simulink model "RadioReceiver_FP_clean"  (R2017a)
settings: Solver=FixedStepDiscrete  StartTime=0.0  StopTime=10.0  RelTol=1e-3
InitFcn:
  | barker = comm.BarkerCode('SamplesPerFrame', 28, 'Length', 11);
  | seq = barker()+1;
  | M = 4;
  | hPSKModTrain   = comm.PSKModulator(M, ...
  |     'PhaseOffset',pi/4, ...
  |     'SymbolMapping','Binary');
  | xPreambleSeq = hPSKModTrain(seq);
  | 
  | 
  | %%%%%%%%%%%%
  | 
  | % AGC Preamble
  | reps = 5;
  | barker = comm.BarkerCode('SamplesPerFrame', 16, 'Length', 13);
  | seq = barker()+1;
  | %preamble = zeros(16*reps,1);
  | preambleFull = repmat(seq,reps,1);
  | rctFilt = comm.RaisedCosineTransmitFilter('FilterSpanInSymbols', 128,...
  | 'RolloffFactor',0.5,...
  | 'OutputSamplesPerSymbol',4);
  | preambleFullFilt = rctFilt(preambleFull);
  | 
  | %%%%%%%%%%%%
  | 
  | RadioSampleRate = 1e6;
  | RadioFrameLength = 1e5;
  | 
  | VibertiTracebackLength = 34+20;
  | numTrainingSamples = 250;
  | crc32Poly = [1 0 0 0 0 0 1 0 0 1 1 0 0 0 0 0 1 0 0 0 1 1 1 0 1 1 0 1 1 0 1 1 1];
  | crcDecodeLag = length(crc32Poly)+2;
  | 
  | %%%%%%%%%%%%
  | 
  | beta = 0.5;
  | span = 8;
  | sps = 4;
  | filterGain = 1;
  | coeff = rcosdesign(beta, span, sps, 'sqrt')*filterGain;
  | 
  | %%%%%%%%%%%%
  | 
  | samplesPerSymbol = 4;
  | maxPacketBits = 8*1500;
  | bItsPerSymbol = 2;
  | CodeRate = 2;
  | tailSymbols = 40;
  | maxPayloadSymbols = maxPacketBits*CodeRate/bItsPerSymbol+tailSymbols;
undefined symbols (not defined in the file or in its folder): F, j
libraries: dsphdlfiltering x20, simulink x7, dspstat3 x2, hdlsllib x2, commdigbbndpm3 x2, commsource2 x1, commcrc2 x1, commseqgen3 x1, commcnvcod2 x1, commutil2 x1, zc706fmc234_lib x1
(part 2 of 3)

== system RadioReceiver_FP_clean/Receiver/Gardner Timing Recovery/Gardner TED Blocks/Real Error ==
  data : Inport
  strobe sum : Inport  Port=2
  Delay : Delay  DelayLength=1
  Product1 : Product  OutDataTypeStr=fixdt(1,16,13)
  Sub : Sum  Inputs=+-  AccumDataTypeStr=fixdt(1,16,13)
  TED Buffer Update1 : Subsystem
  Out1 : Outport
  wires:
  Product1/1 -> Out1/1
  Sub/1 -> Product1/2
  data/1 -> Sub/2, Delay/1
  strobe sum/1 -> TED Buffer Update1/2(strobe sum)
  TED Buffer Update1/2(oldest) -> Sub/1
  Delay/1 -> TED Buffer Update1/1(new data)
  TED Buffer Update1/1(Middle Indx) -> Product1/1

== system RadioReceiver_FP_clean/Receiver/Gardner Timing Recovery/Gardner TED Blocks (NBS)/Imag Error ==
  data : Inport
  strobe sum : Inport  Port=2
  Delay : Delay  DelayLength=1
  Product1 : Product  OutDataTypeStr=fixdt(1,16,13)
  Sub : Sum  Inputs=+-  AccumDataTypeStr=fixdt(1,16,13)
  TED Buffer Update1 : Subsystem
  Out1 : Outport
  wires:
  Product1/1 -> Out1/1
  Sub/1 -> Product1/2
  data/1 -> Sub/2, Delay/1
  strobe sum/1 -> TED Buffer Update1/2(strobe sum)
  TED Buffer Update1/2(oldest) -> Sub/1
  Delay/1 -> TED Buffer Update1/1(new data)
  TED Buffer Update1/1(Middle Indx) -> Product1/1

== system RadioReceiver_FP_clean/Receiver/Gardner Timing Recovery/Gardner TED Blocks (NBS)/Real Error ==
  data : Inport
  strobe sum : Inport  Port=2
  Delay : Delay  DelayLength=1
  Product1 : Product  OutDataTypeStr=fixdt(1,16,13)
  Sub : Sum  Inputs=+-  AccumDataTypeStr=fixdt(1,16,13)
  TED Buffer Update1 : Subsystem
  Out1 : Outport
  wires:
  Product1/1 -> Out1/1
  Sub/1 -> Product1/2
  data/1 -> Sub/2, Delay/1
  strobe sum/1 -> TED Buffer Update1/2(strobe sum)
  TED Buffer Update1/2(oldest) -> Sub/1
  Delay/1 -> TED Buffer Update1/1(new data)
  TED Buffer Update1/1(Middle Indx) -> Product1/1

== system RadioReceiver_FP_clean/Receiver/Gardner Timing Recovery/InterpControl_Blocks/Calculate New mu ==
  W : Inport
  NCOCounter : Inport  Port=2
  Math Reciprocal : Math  Operator=reciprocal  RndMeth=Zero  SaturateOnIntegerOverflow=on
  Product : Product  OutDataTypeStr=fixdt(1,14,15)
  mu : Outport
  wires:
  Product/1 -> mu/1
  W/1 -> Math Reciprocal/1
  Math Reciprocal/1 -> Product/1
  NCOCounter/1 -> Product/2

== system RadioReceiver_FP_clean/Receiver/Frame Sync and Decode/Barker Locate/Measure Phase Ambiguity/Find Max and Set Output Shift ==
  In1 : Inport  OutDataTypeStr=int16
  In2 : Inport  Port=2  OutDataTypeStr=int16
  In4 : Inport  Port=3  OutDataTypeStr=int16
  In5 : Inport  Port=4  OutDataTypeStr=int16
  Enable : EnablePort
  Complex to Real-Imag{,1..3} (4 alike) : ComplexToRealImag  Output=Imag
  Direct Lookup Table (n-D) : LookupNDDirect  NumberOfTableDimensions=1  Table=exp(-(0:pi/2:(pi*3/2)) .* 1i).'  DiagnosticForOutOfRangeInput=Error  TableDataTypeStr=fixdt(1,16,13)
  Maximum : dspstat3/Maximum  operation=maximum  fcn=Index  indexBase=Zero  operateOver=Each column  Dimension=1  InputProcessing=Columns as channels (frame based)  reset=None  roiEnable=off  roiType=Rectangles  roiPortion=Entire ROI  roiOutput=Individual statistics for each ROI  roiFlag=off  roundingMode=Floor  overflowMode=off  accumDataTypeStr=Inherit: Same as product output  accumLastDataTypeStr=Inherit: Same as product output
  Vector Concatenate : Concatenate  NumInputs=4
  Out1 : Outport  InitialOutput=0
  wires:
  Direct Lookup Table (n-D)/1 -> Out1/1
  In1/1 -> Complex to Real-Imag/1
  Complex to Real-Imag2/1 -> Vector Concatenate/3
  Complex to Real-Imag1/1 -> Vector Concatenate/2
  In5/1 -> Complex to Real-Imag3/1
  Complex to Real-Imag3/1 -> Vector Concatenate/4
  Complex to Real-Imag/1 -> Vector Concatenate/1
  Maximum/1 -> Direct Lookup Table (n-D)/1
  In2/1 -> Complex to Real-Imag1/1
  Vector Concatenate/1 -> Maximum/1
  In4/1 -> Complex to Real-Imag2/1

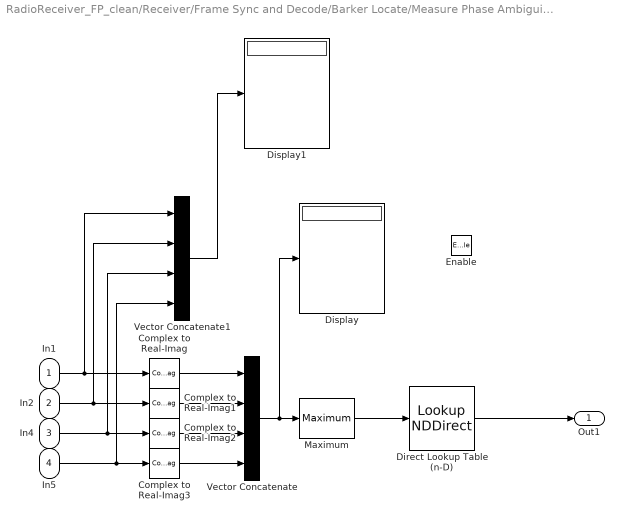
== system RadioReceiver_FP_clean/Receiver/Frame Sync and Decode/Barker Locate/Measure Phase Ambiguity1/Find Max and Set Output Shift ==
  In1 : Inport
  In2 : Inport  Port=2
  In4 : Inport  Port=3
  In5 : Inport  Port=4
  Enable : EnablePort
  Complex to Real-Imag{,1..3} (4 alike) : ComplexToRealImag  Output=Imag
  Direct Lookup Table (n-D) : LookupNDDirect  NumberOfTableDimensions=1  Table=exp(-(0:pi/2:(pi*3/2)) .* 1i).'  DiagnosticForOutOfRangeInput=Error  TableDataTypeStr=fixdt(1,16,13)
  Display : Display
  Display1 : Display
  Maximum : dspstat3/Maximum  operation=maximum  fcn=Index  indexBase=Zero  operateOver=Each column  Dimension=1  InputProcessing=Columns as channels (frame based)  reset=None  roiEnable=off  roiType=Rectangles  roiPortion=Entire ROI  roiOutput=Individual statistics for each ROI  roiFlag=off  roundingMode=Floor  overflowMode=off  accumDataTypeStr=Inherit: Same as product output  accumLastDataTypeStr=Inherit: Same as product output
  Vector Concatenate : Concatenate  NumInputs=4
  Vector Concatenate1 : Concatenate  NumInputs=4
  Out1 : Outport  InitialOutput=0
  wires:
  Direct Lookup Table (n-D)/1 -> Out1/1
  In4/1 -> Vector Concatenate1/3, Complex to Real-Imag2/1
  In2/1 -> Vector Concatenate1/2, Complex to Real-Imag1/1
  In5/1 -> Vector Concatenate1/4, Complex to Real-Imag3/1
  In1/1 -> Vector Concatenate1/1, Complex to Real-Imag/1
  Maximum/1 -> Direct Lookup Table (n-D)/1
  Vector Concatenate/1 -> Display/1, Maximum/1
  Complex to Real-Imag/1 -> Vector Concatenate/1
  Complex to Real-Imag1/1 -> Vector Concatenate/2
  Complex to Real-Imag2/1 -> Vector Concatenate/3
  Complex to Real-Imag3/1 -> Vector Concatenate/4
  Vector Concatenate1/1 -> Display1/1

== system RadioReceiver_FP_clean/Receiver/Frame Sync and Decode/Barker Locate/Measure Phase Ambiguity1/HDL Opt Complex FIR4 ==
  In1 : Inport
  validIn : Inport  Port=2
  Add : Sum  Inputs=+-  AccumDataTypeStr=fixdt(1,16,0)
  Complex to Real-Imag : ComplexToRealImag
  Discrete FIR Filter HDL Optimized : dsphdlfiltering/Discrete FIR Filter HDL Optimized  Numerator=real(Taps)  Sharing=off  SharingFactor=2  SimulateUsing=Code generation  roundingMode=Floor  overflowMode=off  CoefficientsDataTypeStr=Inherit: Same word length as input  CoefficientsMin=[]  CoefficientsMax=[]  OutputDataTypeStr=fixdt(1,16,0)  OutputMin=[]  OutputMax=[]  ValidInPort=on  ReadyPort=off
      settings: SourceProductName=DSP System Toolbox  SourceProductBaseCode=DS
  Discrete FIR Filter HDL Optimized1 : dsphdlfiltering/Discrete FIR Filter HDL Optimized  Numerator=imag(Taps)  Sharing=off  SharingFactor=2  SimulateUsing=Code generation  roundingMode=Floor  overflowMode=off  CoefficientsDataTypeStr=Inherit: Same word length as input  CoefficientsMin=[]  CoefficientsMax=[]  OutputDataTypeStr=fixdt(1,16,0)  OutputMin=[]  OutputMax=[]  ValidInPort=on  ReadyPort=off
      settings: SourceProductName=DSP System Toolbox  SourceProductBaseCode=DS
  Discrete FIR Filter HDL Optimized2 : dsphdlfiltering/Discrete FIR Filter HDL Optimized  Numerator=real(Taps)  Sharing=off  SharingFactor=2  SimulateUsing=Code generation  roundingMode=Floor  overflowMode=off  CoefficientsDataTypeStr=Inherit: Same word length as input  CoefficientsMin=[]  CoefficientsMax=[]  OutputDataTypeStr=fixdt(1,16,0)  OutputMin=[]  OutputMax=[]  ValidInPort=on  ReadyPort=off
      settings: SourceProductName=DSP System Toolbox  SourceProductBaseCode=DS
  Discrete FIR Filter HDL Optimized3 : dsphdlfiltering/Discrete FIR Filter HDL Optimized  Numerator=imag(Taps)  Sharing=off  SharingFactor=2  SimulateUsing=Code generation  roundingMode=Floor  overflowMode=off  CoefficientsDataTypeStr=Inherit: Same word length as input  CoefficientsMin=[]  CoefficientsMax=[]  OutputDataTypeStr=fixdt(1,16,0)  OutputMin=[]  OutputMax=[]  ValidInPort=on  ReadyPort=off
      settings: SourceProductName=DSP System Toolbox  SourceProductBaseCode=DS
  Logical Operator : Logic  Inputs=4  AllPortsSameDT=off  OutDataTypeStr=boolean
  Real-Imag to Complex : RealImagToComplex
  Subtract : Sum  OutDataTypeStr=int16
  Out1 : Outport
  validOut : Outport  Port=2
  wires:
  Discrete FIR Filter HDL Optimized/1 -> Add/1
  Logical Operator/1 -> validOut/1
  Discrete FIR Filter HDL Optimized/2 -> Logical Operator/1
  Discrete FIR Filter HDL Optimized1/2 -> Logical Operator/2
  Discrete FIR Filter HDL Optimized1/1 -> Add/2
  validIn/1 -> Discrete FIR Filter HDL Optimized3/2, Discrete FIR Filter HDL Optimized2/2, Discrete FIR Filter HDL Optimized1/2, Discrete FIR Filter HDL Optimized/2
  In1/1 -> Complex to Real-Imag/1
  Complex to Real-Imag/1 -> Discrete FIR Filter HDL Optimized3/1, Discrete FIR Filter HDL Optimized/1
  Discrete FIR Filter HDL Optimized2/2 -> Logical Operator/3
  Discrete FIR Filter HDL Optimized3/2 -> Logical Operator/4
  Complex to Real-Imag/2 -> Discrete FIR Filter HDL Optimized2/1, Discrete FIR Filter HDL Optimized1/1
  Discrete FIR Filter HDL Optimized2/1 -> Subtract/1
  Discrete FIR Filter HDL Optimized3/1 -> Subtract/2
  Real-Imag to Complex/1 -> Out1/1
  Subtract/1 -> Real-Imag to Complex/2
  Add/1 -> Real-Imag to Complex/1

== system RadioReceiver_FP_clean/Receiver/Frame Sync and Decode/Barker Locate/Measure Phase Ambiguity1/HDL Opt Complex FIR5 ==
  In1 : Inport
  validIn : Inport  Port=2
  Add : Sum  Inputs=+-  AccumDataTypeStr=fixdt(1,16,0)
  Complex to Real-Imag : ComplexToRealImag
  Discrete FIR Filter HDL Optimized : dsphdlfiltering/Discrete FIR Filter HDL Optimized  Numerator=real(Taps)  Sharing=off  SharingFactor=2  SimulateUsing=Code generation  roundingMode=Floor  overflowMode=off  CoefficientsDataTypeStr=Inherit: Same word length as input  CoefficientsMin=[]  CoefficientsMax=[]  OutputDataTypeStr=fixdt(1,16,0)  OutputMin=[]  OutputMax=[]  ValidInPort=on  ReadyPort=off
      settings: SourceProductName=DSP System Toolbox  SourceProductBaseCode=DS
  Discrete FIR Filter HDL Optimized1 : dsphdlfiltering/Discrete FIR Filter HDL Optimized  Numerator=imag(Taps)  Sharing=off  SharingFactor=2  SimulateUsing=Code generation  roundingMode=Floor  overflowMode=off  CoefficientsDataTypeStr=Inherit: Same word length as input  CoefficientsMin=[]  CoefficientsMax=[]  OutputDataTypeStr=fixdt(1,16,0)  OutputMin=[]  OutputMax=[]  ValidInPort=on  ReadyPort=off
      settings: SourceProductName=DSP System Toolbox  SourceProductBaseCode=DS
  Discrete FIR Filter HDL Optimized2 : dsphdlfiltering/Discrete FIR Filter HDL Optimized  Numerator=real(Taps)  Sharing=off  SharingFactor=2  SimulateUsing=Code generation  roundingMode=Floor  overflowMode=off  CoefficientsDataTypeStr=Inherit: Same word length as input  CoefficientsMin=[]  CoefficientsMax=[]  OutputDataTypeStr=fixdt(1,16,0)  OutputMin=[]  OutputMax=[]  ValidInPort=on  ReadyPort=off
      settings: SourceProductName=DSP System Toolbox  SourceProductBaseCode=DS
  Discrete FIR Filter HDL Optimized3 : dsphdlfiltering/Discrete FIR Filter HDL Optimized  Numerator=imag(Taps)  Sharing=off  SharingFactor=2  SimulateUsing=Code generation  roundingMode=Floor  overflowMode=off  CoefficientsDataTypeStr=Inherit: Same word length as input  CoefficientsMin=[]  CoefficientsMax=[]  OutputDataTypeStr=fixdt(1,16,0)  OutputMin=[]  OutputMax=[]  ValidInPort=on  ReadyPort=off
      settings: SourceProductName=DSP System Toolbox  SourceProductBaseCode=DS
  Logical Operator : Logic  Inputs=4  AllPortsSameDT=off  OutDataTypeStr=boolean
  Real-Imag to Complex : RealImagToComplex
  Subtract : Sum  OutDataTypeStr=int16
  Out1 : Outport
  validOut : Outport  Port=2
  wires:
  Discrete FIR Filter HDL Optimized/1 -> Add/1
  Logical Operator/1 -> validOut/1
  Discrete FIR Filter HDL Optimized/2 -> Logical Operator/1
  Discrete FIR Filter HDL Optimized1/2 -> Logical Operator/2
  Discrete FIR Filter HDL Optimized1/1 -> Add/2
  validIn/1 -> Discrete FIR Filter HDL Optimized3/2, Discrete FIR Filter HDL Optimized2/2, Discrete FIR Filter HDL Optimized1/2, Discrete FIR Filter HDL Optimized/2
  In1/1 -> Complex to Real-Imag/1
  Complex to Real-Imag/1 -> Discrete FIR Filter HDL Optimized3/1, Discrete FIR Filter HDL Optimized/1
  Discrete FIR Filter HDL Optimized2/2 -> Logical Operator/3
  Discrete FIR Filter HDL Optimized3/2 -> Logical Operator/4
  Complex to Real-Imag/2 -> Discrete FIR Filter HDL Optimized2/1, Discrete FIR Filter HDL Optimized1/1
  Discrete FIR Filter HDL Optimized2/1 -> Subtract/1
  Discrete FIR Filter HDL Optimized3/1 -> Subtract/2
  Real-Imag to Complex/1 -> Out1/1
  Subtract/1 -> Real-Imag to Complex/2
  Add/1 -> Real-Imag to Complex/1

== system RadioReceiver_FP_clean/Receiver/Frame Sync and Decode/Barker Locate/Measure Phase Ambiguity1/HDL Opt Complex FIR6 ==
  In1 : Inport
  validIn : Inport  Port=2
  Add : Sum  Inputs=+-  AccumDataTypeStr=fixdt(1,16,0)
  Complex to Real-Imag : ComplexToRealImag
  Discrete FIR Filter HDL Optimized : dsphdlfiltering/Discrete FIR Filter HDL Optimized  Numerator=real(Taps)  Sharing=off  SharingFactor=2  SimulateUsing=Code generation  roundingMode=Floor  overflowMode=off  CoefficientsDataTypeStr=Inherit: Same word length as input  CoefficientsMin=[]  CoefficientsMax=[]  OutputDataTypeStr=fixdt(1,16,0)  OutputMin=[]  OutputMax=[]  ValidInPort=on  ReadyPort=off
      settings: SourceProductName=DSP System Toolbox  SourceProductBaseCode=DS
  Discrete FIR Filter HDL Optimized1 : dsphdlfiltering/Discrete FIR Filter HDL Optimized  Numerator=imag(Taps)  Sharing=off  SharingFactor=2  SimulateUsing=Code generation  roundingMode=Floor  overflowMode=off  CoefficientsDataTypeStr=Inherit: Same word length as input  CoefficientsMin=[]  CoefficientsMax=[]  OutputDataTypeStr=fixdt(1,16,0)  OutputMin=[]  OutputMax=[]  ValidInPort=on  ReadyPort=off
      settings: SourceProductName=DSP System Toolbox  SourceProductBaseCode=DS
  Discrete FIR Filter HDL Optimized2 : dsphdlfiltering/Discrete FIR Filter HDL Optimized  Numerator=real(Taps)  Sharing=off  SharingFactor=2  SimulateUsing=Code generation  roundingMode=Floor  overflowMode=off  CoefficientsDataTypeStr=Inherit: Same word length as input  CoefficientsMin=[]  CoefficientsMax=[]  OutputDataTypeStr=fixdt(1,16,0)  OutputMin=[]  OutputMax=[]  ValidInPort=on  ReadyPort=off
      settings: SourceProductName=DSP System Toolbox  SourceProductBaseCode=DS
  Discrete FIR Filter HDL Optimized3 : dsphdlfiltering/Discrete FIR Filter HDL Optimized  Numerator=imag(Taps)  Sharing=off  SharingFactor=2  SimulateUsing=Code generation  roundingMode=Floor  overflowMode=off  CoefficientsDataTypeStr=Inherit: Same word length as input  CoefficientsMin=[]  CoefficientsMax=[]  OutputDataTypeStr=fixdt(1,16,0)  OutputMin=[]  OutputMax=[]  ValidInPort=on  ReadyPort=off
      settings: SourceProductName=DSP System Toolbox  SourceProductBaseCode=DS
  Logical Operator : Logic  Inputs=4  AllPortsSameDT=off  OutDataTypeStr=boolean
  Real-Imag to Complex : RealImagToComplex
  Subtract : Sum  OutDataTypeStr=int16
  Out1 : Outport
  validOut : Outport  Port=2
  wires:
  Discrete FIR Filter HDL Optimized/1 -> Add/1
  Logical Operator/1 -> validOut/1
  Discrete FIR Filter HDL Optimized/2 -> Logical Operator/1
  Discrete FIR Filter HDL Optimized1/2 -> Logical Operator/2
  Discrete FIR Filter HDL Optimized1/1 -> Add/2
  validIn/1 -> Discrete FIR Filter HDL Optimized3/2, Discrete FIR Filter HDL Optimized2/2, Discrete FIR Filter HDL Optimized1/2, Discrete FIR Filter HDL Optimized/2
  In1/1 -> Complex to Real-Imag/1
  Complex to Real-Imag/1 -> Discrete FIR Filter HDL Optimized3/1, Discrete FIR Filter HDL Optimized/1
  Discrete FIR Filter HDL Optimized2/2 -> Logical Operator/3
  Discrete FIR Filter HDL Optimized3/2 -> Logical Operator/4
  Complex to Real-Imag/2 -> Discrete FIR Filter HDL Optimized2/1, Discrete FIR Filter HDL Optimized1/1
  Discrete FIR Filter HDL Optimized2/1 -> Subtract/1
  Discrete FIR Filter HDL Optimized3/1 -> Subtract/2
  Real-Imag to Complex/1 -> Out1/1
  Subtract/1 -> Real-Imag to Complex/2
  Add/1 -> Real-Imag to Complex/1

== system RadioReceiver_FP_clean/Receiver/Frame Sync and Decode/Barker Locate/Measure Phase Ambiguity1/HDL Opt Complex FIR7 ==
  In1 : Inport
  validIn : Inport  Port=2
  Add : Sum  Inputs=+-  AccumDataTypeStr=fixdt(1,16,0)
  Complex to Real-Imag : ComplexToRealImag
  Discrete FIR Filter HDL Optimized : dsphdlfiltering/Discrete FIR Filter HDL Optimized  Numerator=real(Taps)  Sharing=off  SharingFactor=2  SimulateUsing=Code generation  roundingMode=Floor  overflowMode=off  CoefficientsDataTypeStr=Inherit: Same word length as input  CoefficientsMin=[]  CoefficientsMax=[]  OutputDataTypeStr=fixdt(1,16,0)  OutputMin=[]  OutputMax=[]  ValidInPort=on  ReadyPort=off
      settings: SourceProductName=DSP System Toolbox  SourceProductBaseCode=DS
  Discrete FIR Filter HDL Optimized1 : dsphdlfiltering/Discrete FIR Filter HDL Optimized  Numerator=imag(Taps)  Sharing=off  SharingFactor=2  SimulateUsing=Code generation  roundingMode=Floor  overflowMode=off  CoefficientsDataTypeStr=Inherit: Same word length as input  CoefficientsMin=[]  CoefficientsMax=[]  OutputDataTypeStr=fixdt(1,16,0)  OutputMin=[]  OutputMax=[]  ValidInPort=on  ReadyPort=off
      settings: SourceProductName=DSP System Toolbox  SourceProductBaseCode=DS
  Discrete FIR Filter HDL Optimized2 : dsphdlfiltering/Discrete FIR Filter HDL Optimized  Numerator=real(Taps)  Sharing=off  SharingFactor=2  SimulateUsing=Code generation  roundingMode=Floor  overflowMode=off  CoefficientsDataTypeStr=Inherit: Same word length as input  CoefficientsMin=[]  CoefficientsMax=[]  OutputDataTypeStr=fixdt(1,16,0)  OutputMin=[]  OutputMax=[]  ValidInPort=on  ReadyPort=off
      settings: SourceProductName=DSP System Toolbox  SourceProductBaseCode=DS
  Discrete FIR Filter HDL Optimized3 : dsphdlfiltering/Discrete FIR Filter HDL Optimized  Numerator=imag(Taps)  Sharing=off  SharingFactor=2  SimulateUsing=Code generation  roundingMode=Floor  overflowMode=off  CoefficientsDataTypeStr=Inherit: Same word length as input  CoefficientsMin=[]  CoefficientsMax=[]  OutputDataTypeStr=fixdt(1,16,0)  OutputMin=[]  OutputMax=[]  ValidInPort=on  ReadyPort=off
      settings: SourceProductName=DSP System Toolbox  SourceProductBaseCode=DS
  Logical Operator : Logic  Inputs=4  AllPortsSameDT=off  OutDataTypeStr=boolean
  Real-Imag to Complex : RealImagToComplex
  Subtract : Sum  OutDataTypeStr=int16
  Out1 : Outport
  validOut : Outport  Port=2
  wires:
  Discrete FIR Filter HDL Optimized/1 -> Add/1
  Logical Operator/1 -> validOut/1
  Discrete FIR Filter HDL Optimized/2 -> Logical Operator/1
  Discrete FIR Filter HDL Optimized1/2 -> Logical Operator/2
  Discrete FIR Filter HDL Optimized1/1 -> Add/2
  validIn/1 -> Discrete FIR Filter HDL Optimized3/2, Discrete FIR Filter HDL Optimized2/2, Discrete FIR Filter HDL Optimized1/2, Discrete FIR Filter HDL Optimized/2
  In1/1 -> Complex to Real-Imag/1
  Complex to Real-Imag/1 -> Discrete FIR Filter HDL Optimized3/1, Discrete FIR Filter HDL Optimized/1
  Discrete FIR Filter HDL Optimized2/2 -> Logical Operator/3
  Discrete FIR Filter HDL Optimized3/2 -> Logical Operator/4
  Complex to Real-Imag/2 -> Discrete FIR Filter HDL Optimized2/1, Discrete FIR Filter HDL Optimized1/1
  Discrete FIR Filter HDL Optimized2/1 -> Subtract/1
  Discrete FIR Filter HDL Optimized3/1 -> Subtract/2
  Real-Imag to Complex/1 -> Out1/1
  Subtract/1 -> Real-Imag to Complex/2
  Add/1 -> Real-Imag to Complex/1

== system RadioReceiver_FP_clean/Receiver/Frame Sync and Decode/Equalization and Demodulation/DFE/Packeted To Unpacked ==
  In1 : Inport
  Extract Bits : simulink/Logic and Bit Operations/Extract Bits  bitsToExtract=Range of bits  numBits=8  bitIdxRange=[1]  outScalingMode=Treat bit field as an integer
      settings: SourceProductName=Simulink
  Extract Bits1 : simulink/Logic and Bit Operations/Extract Bits  bitsToExtract=Range of bits  numBits=8  bitIdxRange=[0]  outScalingMode=Treat bit field as an integer
      settings: SourceProductName=Simulink
  Vector Concatenate : Concatenate
  Out1 : Outport
  wires:
  In1/1 -> Extract Bits1/1, Extract Bits/1
  Extract Bits/1 -> Vector Concatenate/1
  Extract Bits1/1 -> Vector Concatenate/2
  Vector Concatenate/1 -> Out1/1

== system RadioReceiver_FP_clean/Receiver/Frame Sync and Decode/Equalization and Demodulation/DMA Interface/Convert Payload Length To Bytes ==
  In1 : Inport
  Constant : Constant  Value=uint16(32-1)  SampleTime=-1
  Data Type Conversion : DataTypeConversion  OutDataTypeStr=uint32
  Remove CRC Length : Sum  Inputs=+-  AccumDataTypeStr=uint16
  Shift Arithmetic1 : ArithShift  BitShiftNumber=3  BitShiftDirection=Right
  Shift Arithmetic2 : ArithShift  BitShiftNumber=1  BitShiftDirection=Right
  Out1 : Outport
  wires:
  In1/1 -> Shift Arithmetic2/1
  Remove CRC Length/1 -> Shift Arithmetic1/1
  Shift Arithmetic2/1 -> Remove CRC Length/1
  Shift Arithmetic1/1 -> Data Type Conversion/1
  Constant/1 -> Remove CRC Length/2
  Data Type Conversion/1 -> Out1/1

== system RadioReceiver_FP_clean/Receiver/Frame Sync and Decode/Equalization and Demodulation/Descramble and Decode/2 Bit Descrambler ==
  note: This is a special Descrambler which can process 2 bits at a time
  u1 : Inport
  reset : Inport  Port=2
  Demux1 : Demux  Outputs=2
  MATLAB Function : MATLAB Function  TreatAsAtomicUnit=on
  Mux : Mux  Inputs=2
  Selector1 : Selector  IndexOptions=Index vector (dialog)  Indices=find(polynom(2:end))  OutputSizes=1
  Selector2 : Selector  IndexOptions=Index vector (dialog)  Indices=find(polynom(2:end))  OutputSizes=1
  input_xor1 : Logic  Operator=XOR  IconShape=distinctive  AllPortsSameDT=off  OutDataTypeStr=boolean
  input_xor2 : Logic  Operator=XOR  IconShape=distinctive  AllPortsSameDT=off  OutDataTypeStr=boolean
  state_xor1 : Logic  Operator=XOR  Inputs=1  IconShape=distinctive  AllPortsSameDT=off  OutDataTypeStr=boolean
  state_xor2 : Logic  Operator=XOR  Inputs=1  IconShape=distinctive  AllPortsSameDT=off  OutDataTypeStr=boolean
  y1 : Outport  InitialOutput=0
  wires:
  u1/1 -> Demux1/1, MATLAB Function/1(bits)
  reset/1 -> MATLAB Function/2(reset)
  MATLAB Function/1(bufferA) -> Selector1/1
  MATLAB Function/2(bufferB) -> Selector2/1
  Mux/1 -> y1/1
  state_xor1/1 -> input_xor1/1
  state_xor2/1 -> input_xor2/1
  input_xor2/1 -> Mux/2
  input_xor1/1 -> Mux/1
  Selector1/1 -> state_xor1/1
  Selector2/1 -> state_xor2/1
  Demux1/1 -> input_xor1/2
  Demux1/2 -> input_xor2/2  "data_in"

== system RadioReceiver_FP_clean/Receiver/Frame Sync and Decode/Equalization and Demodulation/Descramble and Decode/Enabled Subsystem ==
  In1 : Inport
  Enable : EnablePort
  To Workspace : ToWorkspace  VariableName=crcConditions  SaveFormat=Structure  SampleTime=-1
  wires:
  In1/1 -> To Workspace/1

== system RadioReceiver_FP_clean/Receiver/Gardner Timing Recovery/Gardner TED Blocks/Imag Error/TED Buffer Update1 ==
  new data : Inport
  strobe sum : Inport  Port=2
  Delay{,1..3} (4 alike) : Delay  DelayLength=1
  Multiport Switch{,1..3} (4 alike) : MultiPortSwitch  DataPortOrder=Zero-based contiguous  DataPortIndices={0,1,[2,3]}
  Zero bit : Constant  Value=0  OutDataTypeStr=fixdt(1,16,13)  SampleTime=1e-6
  Middle Indx : Outport
  oldest : Outport  Port=2
  wires:
  strobe sum/1 -> Multiport Switch3/1, Multiport Switch2/1, Multiport Switch1/1, Multiport Switch/1
  Delay/1 -> Multiport Switch/2
  Delay1/1 -> Multiport Switch/3, Multiport Switch1/2
  Delay2/1 -> Multiport Switch/4, Multiport Switch1/3, Multiport Switch2/2
  new data/1 -> Multiport Switch3/4, Multiport Switch3/3
  Zero bit/1 -> Multiport Switch2/4
  Delay3/1 -> Multiport Switch1/4, Multiport Switch2/3, Multiport Switch3/2
  Multiport Switch1/1 -> Delay1/1
  Multiport Switch2/1 -> Middle Indx/1, Delay2/1
  Multiport Switch3/1 -> Delay3/1
  Multiport Switch/1 -> Delay/1, oldest/1

== system RadioReceiver_FP_clean/Receiver/Gardner Timing Recovery/Gardner TED Blocks/Real Error/TED Buffer Update1 ==
  new data : Inport
  strobe sum : Inport  Port=2
  Delay{,1..3} (4 alike) : Delay  DelayLength=1
  Multiport Switch{,1..3} (4 alike) : MultiPortSwitch  DataPortOrder=Zero-based contiguous  DataPortIndices={0,1,[2,3]}
  Zero bit : Constant  Value=0  OutDataTypeStr=fixdt(1,16,13)  SampleTime=1e-6
  Middle Indx : Outport
  oldest : Outport  Port=2
  wires:
  strobe sum/1 -> Multiport Switch3/1, Multiport Switch2/1, Multiport Switch1/1, Multiport Switch/1
  Delay/1 -> Multiport Switch/2
  Delay1/1 -> Multiport Switch/3, Multiport Switch1/2
  Delay2/1 -> Multiport Switch/4, Multiport Switch1/3, Multiport Switch2/2
  new data/1 -> Multiport Switch3/4, Multiport Switch3/3
  Zero bit/1 -> Multiport Switch2/4
  Delay3/1 -> Multiport Switch1/4, Multiport Switch2/3, Multiport Switch3/2
  Multiport Switch1/1 -> Delay1/1
  Multiport Switch2/1 -> Middle Indx/1, Delay2/1
  Multiport Switch3/1 -> Delay3/1
  Multiport Switch/1 -> Delay/1, oldest/1

== system RadioReceiver_FP_clean/Receiver/Gardner Timing Recovery/Gardner TED Blocks (NBS)/Imag Error/TED Buffer Update1 ==
  new data : Inport
  strobe sum : Inport  Port=2
  Delay{,1..3} (4 alike) : Delay  DelayLength=1
  Multiport Switch{,1..3} (4 alike) : MultiPortSwitch  DataPortOrder=Zero-based contiguous  DataPortIndices={0,1,[2,3]}
  Zero bit : Constant  Value=0  OutDataTypeStr=fixdt(1,16,13)  SampleTime=1e-6
  Middle Indx : Outport
  oldest : Outport  Port=2
  wires:
  strobe sum/1 -> Multiport Switch3/1, Multiport Switch2/1, Multiport Switch1/1, Multiport Switch/1
  Delay/1 -> Multiport Switch/2
  Delay1/1 -> Multiport Switch/3, Multiport Switch1/2
  Delay2/1 -> Multiport Switch/4, Multiport Switch1/3, Multiport Switch2/2
  new data/1 -> Multiport Switch3/4, Multiport Switch3/3
  Zero bit/1 -> Multiport Switch2/4
  Delay3/1 -> Multiport Switch1/4, Multiport Switch2/3, Multiport Switch3/2
  Multiport Switch1/1 -> Delay1/1
  Multiport Switch2/1 -> Middle Indx/1, Delay2/1
  Multiport Switch3/1 -> Delay3/1
  Multiport Switch/1 -> Delay/1, oldest/1

== system RadioReceiver_FP_clean/Receiver/Gardner Timing Recovery/Gardner TED Blocks (NBS)/Real Error/TED Buffer Update1 ==
  new data : Inport
  strobe sum : Inport  Port=2
  Delay{,1..3} (4 alike) : Delay  DelayLength=1
  Multiport Switch{,1..3} (4 alike) : MultiPortSwitch  DataPortOrder=Zero-based contiguous  DataPortIndices={0,1,[2,3]}
  Zero bit : Constant  Value=0  OutDataTypeStr=fixdt(1,16,13)  SampleTime=1e-6
  Middle Indx : Outport
  oldest : Outport  Port=2
  wires:
  strobe sum/1 -> Multiport Switch3/1, Multiport Switch2/1, Multiport Switch1/1, Multiport Switch/1
  Delay/1 -> Multiport Switch/2
  Delay1/1 -> Multiport Switch/3, Multiport Switch1/2
  Delay2/1 -> Multiport Switch/4, Multiport Switch1/3, Multiport Switch2/2
  new data/1 -> Multiport Switch3/4, Multiport Switch3/3
  Zero bit/1 -> Multiport Switch2/4
  Delay3/1 -> Multiport Switch1/4, Multiport Switch2/3, Multiport Switch3/2
  Multiport Switch1/1 -> Delay1/1
  Multiport Switch2/1 -> Middle Indx/1, Delay2/1
  Multiport Switch3/1 -> Delay3/1
  Multiport Switch/1 -> Delay/1, oldest/1

== matlab function RadioReceiver_FP_clean/Receiver/Frame Sync and Decode/Equalization and Demodulation/CRC Check/Check CRC Result (DEBUG) ==
  data: bits input; start input; done input; valid input; err input
function fcn(bits, start, done, valid, err)

persistent buffer

if isempty(buffer)
    buffer = fi(false(1032,1),0,1,0);
end

buffer = [buffer(2:end);bits];

if done && valid
    if err
        fprintf('CRC Error (HDL CRC)\n');
    else
        fprintf('CRC Passed (HDL CRC)\n');
    end
end
if err % Flag if any error every occurs
    fprintf('CRC Error Type 2 (HDL CRC)\n');
end

== matlab function RadioReceiver_FP_clean/Receiver/Gardner Timing Recovery/Gardner TED/Gardner TED ==
  data: u input; strobe input; e output
% function e = TED(u,strobe)
% 
% persistent TEDBuffer StrobeHistory t1Indx t2Indx
% 
% if isempty(TEDBuffer)
%     samplesPerSymbol = 4;
%     TEDBuffer = complex(zeros(samplesPerSymbol,1));
%     StrobeHistory = false(samplesPerSymbol,1);
%     %rem(samplesPerSymbol,2);
%     REM_SPS_2 = 0;
%     t1Indx = (samplesPerSymbol/2 + 1 - REM_SPS_2);
%     t2Indx = (samplesPerSymbol/2 + 1);
% end
% 
% % Determine timing error
% if strobe && all(~StrobeHistory(2:end))
%     midSampleAverage = (TEDBuffer(t1Indx) + TEDBuffer(t2Indx))/2;
%     e = real(midSampleAverage) * (real(TEDBuffer(1)) - real(u)) + ...;
%         imag(midSampleAverage) * (imag(TEDBuffer(1)) - imag(u));
% else
%     e = 0;
% end
% 
% % Compensate for bit slips by bit stuffing
% switch sum([StrobeHistory(2:end); strobe])
%     case 0
%         % Skip current sample if NO strobe across N samples, i.e.,
%         % StrobeHistory(2:end) = [0, 0, ..., 0] & strobe = 0
%     case 1
%         % Shift TED buffer regularly if ONE strobe across N samples, i.e.,
%         TEDBuffer = [TEDBuffer(2:end); u];
%     otherwise % > 1
%         % Stuff a missing sample if TWO strobes across N samples, i.e.,
%         % StrobeHistory(2:end) = [1, 0, ..., 0] & strobe = 1
%         TEDBuffer = [TEDBuffer(3:end); 0; u];
%         
% end  % End of TED
% 
% 
% % Update strobe history
% StrobeHistory = [StrobeHistory(2:end); strobe];

function e = TED(u,strobe)

persistent TEDBufferR TEDBufferI StrobeHistory

WL = uint8(16);
FL = uint8(13);
fm = fimath('RoundingMethod', 'Floor',...
    'OverflowAction', 'Wrap',...
    'ProductMode','FullPrecision',...
    'MaxProductWordLength', 128,...
    'SumMode','FullPrecision',...
    'MaxSumWordLength', 128);
%u = fi(u, 1, WL, FL, fm);

% Constants
samplesPerSymbol = uint8(4);
middleIndx = uint8(3);

% Async
if isempty(TEDBufferR)
    TEDBufferR = fi(zeros(samplesPerSymbol,1), 1, WL, FL, fm);
    TEDBufferI = fi(zeros(samplesPerSymbol,1), 1, WL, FL, fm);
    StrobeHistory = false(samplesPerSymbol,1);
end

s = uint8(StrobeHistory(2)) + uint8(StrobeHistory(3)) +...
    uint8(StrobeHistory(4)) + uint8(strobe);
ur = real(u);
ui = imag(u);

% Determine timing error
if strobe && (s==uint8(1)) 
    e = fi(...
        TEDBufferR(middleIndx)*( TEDBufferR(1) - ur ) + ...
        TEDBufferI(middleIndx)*( TEDBufferI(1) - ui ),...
        1, 16, 11, fm);    
else
    e = fi(0, 1, 16, 11, fm);
end

% Compensate for bit slips by bit stuffing
switch s
    case uint8(0)
        % Skip current sample if NO strobe across N samples, i.e.,
        % StrobeHistory(2:end) = [0, 0, ..., 0] & strobe = 0
    case uint8(1)
        % Shift TED buffer regularly if ONE strobe across N samples, i.e.,
        TEDBufferR = [TEDBufferR(2:samplesPerSymbol); ur];
        TEDBufferI = [TEDBufferI(2:samplesPerSymbol); ui];
    otherwise % > 1
        % Stuff a missing sample if TWO strobes across N samples, i.e.,
        % StrobeHistory(2:end) = [1, 0, ..., 0] & strobe = 1
        TEDBufferR = [TEDBufferR(3:samplesPerSymbol); 0; ur];
        TEDBufferI = [TEDBufferI(3:samplesPerSymbol); 0; ui];
        
end  % End of TED

% Save history
StrobeHistory = [StrobeHistory(2:samplesPerSymbol); strobe];

== matlab function RadioReceiver_FP_clean/Receiver/Frame Sync and Decode/Equalization and Demodulation/Header Controller ==
  data: headerStart input; enableDownstream output; packetLenBitsOut output; data input; resetViterbi output; crcStart output
function [enableDownstream,packetLenBitsOut,resetViterbi,crcStart] = EvalHeader(headerStart, data)

persistent counter sum1 sum2 packetLenBits lastMode savedPacketLenBits

% The header contains 16 bits, but each bit is duplicated to make checking
% easier

% Note this block works on symbols (2bits) but 1 symbol -> 1 decoded bit

% PacketLength = (Data+CRC+40(TB)+68)/CodeRate

% NOTE TAIL BITS HERE ARE REALLY USED TO DEAL WITH VITERBI LAG SO:
% TailBitsWithLagPadding > TracebackLength

%% Constants
numHeaderBits = uint8(16); % Header is this many bits
powersOfTwo = uint32([1 2 4 8 16 32 64 128 256 512 1024 2048 4096 8192 16384 32768]);
%TracebackLength = uint32(34)+uint32(20);
%CRCLen = uint32(32);
CodeRateINV = uint32(2);%1/CodeRate;
TailBitsWithLagPadding = uint32(uint32(40)+34*2+1);
% Flag when CRC porition of packet starts relative to header
%crcSignalStartLocation = uint32((TailBitsWithLagPadding+CRCLen)*CodeRateINV); % Must be even
crcSignalStartLocation = uint32((TailBitsWithLagPadding)*CodeRateINV); % Must be even

% Async
if isempty(counter)
    packetLenBits = uint32(0);
    sum1 = uint32(0);
    sum2 = uint32(0);
    counter = uint8(numHeaderBits);
    lastMode = uint8(3);
    savedPacketLenBits = uint16(0);
end

%% Sync
% Got a header now enable certain mode
if headerStart
    mode = uint8(0);
else
    mode = lastMode;
end

switch mode
    %% Reset on preamble flag and setup for header processing
    case uint8(0)
        crcStart = false;
        resetViterbi = false;
        enableDownstream = false;
        sum1 = uint32(0);
        sum2 = uint32(0);
        counter = uint8(1);
        lastMode = uint8(1); % Go to next state
        packetLenBitsOut = uint16(0);
        
    %% Process header
    case 1 
        crcStart = false;
        enableDownstream = false; %%%%%%%%%%% CHECK!
        
        % Convert header bits (bit by bit)
        if data(1)
            sum1 = sum1 + powersOfTwo(counter);
        end
        if data(2)
            sum2 = sum2 + powersOfTwo(counter);
        end
        counter = counter + uint8(1);
        
        if counter>numHeaderBits
            % Check header
            if sum1~=sum2 % Fail
                packetLenBits = uint32(0);
                lastMode = uint8(3);
                resetViterbi = false;
                packetLenBitsOut = uint16(0);
                savedPacketLenBits = uint16(0);
%                 fprintf('Header Check failed (possible false detection)\n');
            else % Pass
                % Saved header info and trigger downstream
                packetLenBits = uint32(sum1);
                lastMode = uint8(2);
                resetViterbi = true;
                packetLenBitsOut = uint16(sum1-crcSignalStartLocation);
                savedPacketLenBits = uint16(sum1-crcSignalStartLocation);
%                 fprintf('Header Found | Packet is %d bits long\n',int32(sum1));            
            end
        else
            packetLenBitsOut = uint16(0);
            resetViterbi = false;
        end
        
    %% Decrement sample counter
    case 2 
        resetViterbi = false;
        crcStart = (packetLenBits==crcSignalStartLocation);
        if packetLenBits>uint32(0)
            enableDownstream = true;
            packetLenBits = packetLenBits - uint32(2); % We get 2 bits each call
            packetLenBitsOut = savedPacketLenBits;
        else
            enableDownstream = false;
            lastMode = uint8(3);
            packetLenBitsOut = uint16(0); %Reset
            savedPacketLenBits = uint16(0);%Reset
        end
            
    %% Not processing anything
    otherwise % mode>2
        crcStart = false;
        resetViterbi = false;
        enableDownstream = false;
        packetLenBitsOut = uint16(0);
end

%%

% % Set default flags, which may change
% resetViterbi = false;
% crcStart = false;
% 
% % Reset when preamble found (barker sequence)
% if headerStart
%     sum1 = uint32(0);
%     sum2 = uint32(0);
%     counter = uint32(1);
% end
% 
% % Send data downstream to
% enableDownstream = packetLenBits>uint32(0);
% 
% % Flag when we are in CRC section of packet
% % Enable signal will relate to first bit of CRC portion of packet
% if packetLenBits==crcSignalStartLocation
%     crcStart = true;
% end
% 
% % Decrement packet length counter
% if enableDownstream
%     packetLenBits = packetLenBits - uint32(2); % Get 2 bits each call
% end
% 
% % Process header
% if counter<=headerBits
%     % Convert header bits (bit by bit)
%     if data(1)
%         sum1 = sum1 + powersOfTwo(counter);
%     end
%     if data(2)
%         sum2 = sum2 + powersOfTwo(counter);
%     end
%     counter = counter + uint32(1);
%     
%     if counter>headerBits
%         % Check header
%         if sum1~=sum2
%             packetLenBits = uint32(0);
%             enableDownstream = false;
%             fprintf('Header Check failed (possible false detection)\n');
%         else
%             % Saved header info and trigger downstream
%             packetLenBits = uint32(sum1);
%             fprintf('Header Found | Packet is %d bits long\n',int32(sum1));
%             resetViterbi = true;
%             enableDownstream = true;
%         end
%     end
%     
% end

== matlab function RadioReceiver_FP_clean/Receiver/Gardner Timing Recovery/InterControl/InterControl ==
  data: v input; strobe output; Mu output
% function [strobe,Mu] = InterpolationControl(v)
% 
% persistent NCOCounter samplesPerSymbol MuS
% if isempty(NCOCounter)
%     NCOCounter = 0;
%     samplesPerSymbol = 4;
%     MuS = complex(0);
% end
%     
% W = v + 1/samplesPerSymbol;
% % Check strobe condition
% strobe = NCOCounter < W;
% if strobe
%     Mu = complex(NCOCounter/W); % Update factional interval
%     MuS = Mu;
% else
%     Mu = MuS;
% end
% % Decrement counter
% NCOCounter = mod(NCOCounter-W,1);

% function [strobe,Mu] = InterpolationControl(v)
% 
% persistent NCOCounter MuS
% 
% %v = fi(v,1,16,20);
% 
% samplesPerSymbol = fi(4,0,4,1);
% 
% if isempty(NCOCounter)
%     NCOCounter = fi(v,0,16,16);
%     MuS = fi(complex(0),0,16,16);
% end
%     
% W = fi(v + 1/samplesPerSymbol,0,16,17);
%     
% % Check strobe condition
% strobe = NCOCounter < W;
% if strobe
%     Mu = fi(complex(NCOCounter/W),0,16,16); % Update factional interval
%     MuS = Mu;
% else
%     Mu = MuS;
% end
% % Decrement counter
% NCOmW = fi(NCOCounter-W,1,16,15);
% 
% % Exceeding Modulus cases
% if (NCOmW>fi(1,0,1,0)) % Modulus catch
%     NCOCounter = fi(NCOmW-fi(1,0,1,0),0,16,16);
% elseif (NCOmW<fi(-1,1,2,0)) % Modulus catch
%     NCOCounter = fi(-1*(NCOmW+fi(1,0,1,0)),0,16,16);
% % ABS only cases
% elseif (NCOmW<fi(0,0,1,1)) % negative
%     NCOCounter = fi(-1*NCOmW,0,16,16);
% else
%     NCOCounter = fi(NCOmW,0,16,16);
% end

%auto-generated
%#codegen
function [strobe,Mu] = InterpolationControl(v)

fm = get_fimath();
v = fi(v, 1, 16, 20, fm);

persistent NCOCounter samplesPerSymbol MuS
if isempty(NCOCounter)
    NCOCounter = fi(0, 0, 16, 16, fm);
    samplesPerSymbol = fi(4, 0, 16, 13, fm);
    MuS = fi(complex(0), 0, 16, 16, fm);
end
    
W = fi(v + fi_div(fi(1, 0, 1, 0, fm), samplesPerSymbol), 0, 16, 17, fm);
% Check strobe condition
strobe = NCOCounter < W;
if strobe
    Mu = fi(complexx(fi_div(NCOCounter, W)), 0, 16, 16, fm); % Update factional interval
    MuS(:) = Mu;
else
    Mu = fi(MuS, 0, 16, 16, fm);
end
% Decrement counter
%NCOCounter(:) = mod(fi_signed(NCOCounter)-W,fi(1, 0, 1, 0, fm));
NCOCounter(:) = fi_signed(NCOCounter)-W;
end



function c = complexx(varargin)
    coder.inline( 'always' );
    if nargin==2
        re = varargin{ 1 };
        im = varargin{ 2 };
        if isfi( re ) && isfi( im )
            % Choose wider type
            NT = fixed.aggregateType( re, im );
            c = complex( fi( re, NT ), fi( im, NT ) );
        else
            c = complex( re, im );
        end
    elseif nargin==1
        c = complex( varargin{ 1 } );
    end
end


function ntype = divideType(a,b)
    coder.inline( 'always' );
    nt1 = numerictype( a );
    nt2 = numerictype( b );
    maxFL = max( [ min( nt1.WordLength, nt1.FractionLength ), min( nt2.WordLength, nt2.FractionLength ) ] );
    FL = max( maxFL, 24 );
    extraBits = (FL - maxFL);
    WL = nt1.WordLength + nt2.WordLength;
    WL = min( WL, 124 );
    if (WL + extraBits)<64
        ntype = numerictype( nt1.Signed || nt2.Signed, WL + extraBits, FL );
    else
        ntype = numerictype( nt1.Signed || nt2.Signed, WL, FL );
    end
end


function c = fi_div(a,b)
    coder.inline( 'always' );
    if isfi( a ) && isfi( b ) && isscalar( b )
        a1 = fi( a, 'RoundMode', 'fix' );
        b1 = fi( b, 'RoundMode', 'fix' );
        c1 = divide( divideType( a1, b1 ), a1, b1 );
        c = fi( c1, numerictype( c1 ), fimath( a ) );
    else
        c = a/b;
    end
end


function y = fi_signed(a)
    coder.inline( 'always' );
    if isfi( a ) && ~(issigned( a ))
        nt = numerictype( a );
        new_nt = numerictype( 1, nt.WordLength + 1, nt.FractionLength );
        y = fi( a, new_nt, fimath( a ) );
    else
        y = a;
    end
end

function fm = get_fimath()
	fm = fimath('RoundingMethod', 'Floor',...
	     'OverflowAction', 'Wrap',...
	     'ProductMode','FullPrecision',...
	     'MaxProductWordLength', 128,...
	     'SumMode','FullPrecision',...
	     'MaxSumWordLength', 128);
end

== matlab function RadioReceiver_FP_clean/Receiver/Gardner Timing Recovery/InterControl/InterControl_FixPt ==
  settings: fimath=fimath('RoundingMethod', 'Floor', 'OverflowAction', 'Wrap', 'ProductMode', 'FullPrecision', 'MaxProductWordLength', 128, 'SumMode', 'FullPrecision', 'MaxSumWordLength', 128)
  data: v input; strobe output; Mu output
%auto-generated
%#codegen
function [strobe,Mu] = InterpolationControl_fixpt(v)

fm = get_fimath();
v = fi(v, 1, 16, 20, fm);

persistent NCOCounter samplesPerSymbol MuS
if isempty(NCOCounter)
    NCOCounter = fi(0, 0, 16, 16, fm);
    samplesPerSymbol = fi(4, 0, 16, 13, fm);
    MuS = fi(complex(0), 0, 16, 16, fm);
end
    
W = fi(v + fi_div(fi(1, 0, 1, 0, fm), samplesPerSymbol), 0, 16, 17, fm);
% Check strobe condition
strobe = NCOCounter < W;
if strobe
    Mu = fi(complexx(fi_div(NCOCounter, W)), 0, 16, 16, fm); % Update factional interval
    MuS(:) = Mu;
else
    Mu = fi(MuS, 0, 16, 16, fm);
end
% Decrement counter
NCOCounter(:) = mod(fi_signed(NCOCounter)-W,fi(1, 0, 1, 0, fm));
end



function c = complexx(varargin)
    coder.inline( 'always' );
    if nargin==2
        re = varargin{ 1 };
        im = varargin{ 2 };
        if isfi( re ) && isfi( im )
            % Choose wider type
            NT = fixed.aggregateType( re, im );
            c = complex( fi( re, NT ), fi( im, NT ) );
        else
            c = complex( re, im );
        end
    elseif nargin==1
        c = complex( varargin{ 1 } );
    end
end


function ntype = divideType(a,b)
    coder.inline( 'always' );
    nt1 = numerictype( a );
    nt2 = numerictype( b );
    maxFL = max( [ min( nt1.WordLength, nt1.FractionLength ), min( nt2.WordLength, nt2.FractionLength ) ] );
    FL = max( maxFL, 24 );
    extraBits = (FL - maxFL);
    WL = nt1.WordLength + nt2.WordLength;
    WL = min( WL, 124 );
    if (WL + extraBits)<64
        ntype = numerictype( nt1.Signed || nt2.Signed, WL + extraBits, FL );
    else
        ntype = numerictype( nt1.Signed || nt2.Signed, WL, FL );
    end
end


function c = fi_div(a,b)
    coder.inline( 'always' );
    if isfi( a ) && isfi( b ) && isscalar( b )
        a1 = fi( a, 'RoundMode', 'fix' );
        b1 = fi( b, 'RoundMode', 'fix' );
        c1 = divide( divideType( a1, b1 ), a1, b1 );
        c = fi( c1, numerictype( c1 ), fimath( a ) );
    else
        c = a/b;
    end
end


function y = fi_signed(a)
    coder.inline( 'always' );
    if isfi( a ) && ~(issigned( a ))
        nt = numerictype( a );
        new_nt = numerictype( 1, nt.WordLength + 1, nt.FractionLength );
        y = fi( a, new_nt, fimath( a ) );
    else
        y = a;
    end
end

function fm = get_fimath()
	fm = fimath('RoundingMethod', 'Floor',...
	     'OverflowAction', 'Wrap',...
	     'ProductMode','FullPrecision',...
	     'MaxProductWordLength', 128,...
	     'SumMode','FullPrecision',...
	     'MaxSumWordLength', 128);
end

== matlab function RadioReceiver_FP_clean/Receiver/Gardner Timing Recovery/Gardner TED/Gardner TED_FixPt ==
  settings: fimath=fimath('RoundingMethod', 'Floor', 'OverflowAction', 'Wrap', 'ProductMode', 'FullPrecision', 'MaxProductWordLength', 128, 'SumMode', 'FullPrecision', 'MaxSumWordLength', 128)
  data: u input; strobe input; e output
%auto-generated
%#codegen
function e = TED_fixpt(u,strobe)

fm = get_fimath();
u = fi(u, 1, 16, 13, fm);

persistent TEDBuffer StrobeHistory t1Indx t2Indx

if isempty(TEDBuffer)
    samplesPerSymbol = fi(4, 0, 16, 13, fm);
    TEDBuffer = fi(complex(zeros(fi_toint(samplesPerSymbol),1)), 1, 16, 13, fm);
    StrobeHistory = false(fi_toint(samplesPerSymbol),1);
    %rem(samplesPerSymbol,2);
    REM_SPS_2 = fi(0, 1, 16, 4, fm);
    t1Indx = fi((fi_div_by_shift(samplesPerSymbol, 1) + fi(1, 0, 1, 0, fm) - REM_SPS_2), 0, 16, 14, fm);
    t2Indx = fi((fi_div_by_shift(samplesPerSymbol, 1) + fi(1, 0, 1, 0, fm)), 0, 16, 14, fm);
end

% Determine timing error
if strobe && all(~StrobeHistory(2:end))
    midSampleAverage = fi(fi_div_by_shift((TEDBuffer(t1Indx) + TEDBuffer(t2Indx)), 1), 1, 16, 13, fm);
    e = fi(real(midSampleAverage) * (fi_signed(real(TEDBuffer(1))) - real(u)) + ...;
        imag(midSampleAverage) * (fi_signed(imag(TEDBuffer(1))) - imag(u)), 1, 16, 11, fm);
else
    e = fi(0, 1, 16, 11, fm);
end

% Compensate for bit slips by bit stuffing
switch sum([StrobeHistory(2:end); strobe])
    case fi(0, 0, 1, 0, fm)
        % Skip current sample if NO strobe across N samples, i.e.,
        % StrobeHistory(2:end) = [0, 0, ..., 0] & strobe = 0
    case fi(1, 0, 1, 0, fm)
        % Shift TED buffer regularly if ONE strobe across N samples, i.e.,
        TEDBuffer(:) = [fi(TEDBuffer(2:end), 1, 16, 13, fm); u];
    otherwise % > 1
        % Stuff a missing sample if TWO strobes across N samples, i.e.,
        % StrobeHistory(2:end) = [1, 0, ..., 0] & strobe = 1
        TEDBuffer(:) = [fi(TEDBuffer(3:end), 1, 16, 13, fm); fi(0, 0, 1, 0, fm); u];
        
end  % End of TED


% Update strobe history
StrobeHistory(:) = [StrobeHistory(2:end); strobe];
end



function y = fi_div_by_shift(a,shift_len)
    coder.inline( 'always' );
    if isfi( a )
        nt = numerictype( a );
        fm = fimath( a );
        nt_bs = numerictype( nt.Signed, nt.WordLength + shift_len, nt.FractionLength + shift_len );
        y = bitsra( fi( a, nt_bs, fm ), shift_len );
    else
        y = a/2^shift_len;
    end
end


function y = fi_signed(a)
    coder.inline( 'always' );
    if isfi( a ) && ~(issigned( a ))
        nt = numerictype( a );
        new_nt = numerictype( 1, nt.WordLength + 1, nt.FractionLength );
        y = fi( a, new_nt, fimath( a ) );
    else
        y = a;
    end
end


function y = fi_toint(u)
    coder.inline( 'always' );
    if isfi( u )
        nt = numerictype( u );
        s = nt.SignednessBool;
        wl = nt.WordLength;
        y = int32( fi( u, s, wl, 0, hdlfimath ) );
    else
        y = int32( u );
    end
end

function fm = get_fimath()
	fm = fimath('RoundingMethod', 'Floor',...
	     'OverflowAction', 'Wrap',...
	     'ProductMode','FullPrecision',...
	     'MaxProductWordLength', 128,...
	     'SumMode','FullPrecision',...
	     'MaxSumWordLength', 128);
end

== matlab function RadioReceiver_FP_clean/Receiver/Frequency Recovery/Loop Filter/Flip Sign ==
  data: u input; y output
function y = fcn(u)

WL = 25;
FP = 20;

% Flip sign x = (~y) + 1
u8 = bitcmp(int8(u));
y = fi(u8+int8(1),1,WL,FP);

== matlab function RadioReceiver_FP_clean/Receiver/Frame Sync and Decode/Enable Equalizer and Packet Decode ==
  data: eof input; start input; enable output
function enable = Counter(eof,start)

persistent count maxCount lastEOF

if isempty(count)
    count = uint32(0);
    maxCount = uint32(2^16); % Largest possible packet length
    lastEOF = false;
end

% Got a barker preamble start allowing data into equalizer
if start
    count = maxCount;
end

% Check on change from true to false
if lastEOF && ~eof
%     fprintf('Frame end reached\n');
    count = uint32(0);
end
lastEOF = eof;

% Past end of max frame size
if count>0
    count = count - uint32(1);
end

% Enable downstream
enable = count>uint32(0);
